simulink model "elevator"  (Simulink 6.5)
settings: Solver=FixedStepDiscrete  StartTime=0.0  StopTime=inf  FixedStep=0.01  RelTol=1e-3
settings Model: Creator=sja  LastModifiedBy=haf  ExtModeAutoUpdateStatusClock=off
settings DebuggingCC: MultiTaskDSMMsg=warning  MultiTaskCondExecSysMsg=none  StrictBusMsg=None
settings RTWCC: IncludeERTFirstTime=on

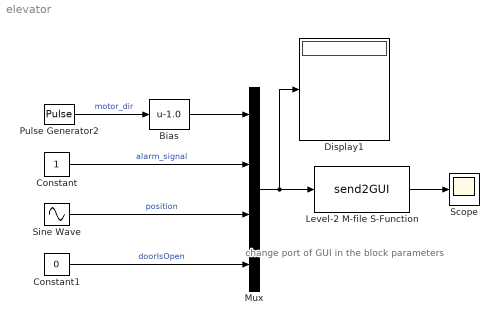
== system elevator ==
  note: change port of
      | GUI in the block
      | parameters
  Bias : Bias  Bias=-1.0
  Constant : Constant  Value=1  OutDataType=sfix(16)  ConRadixGroup=Use specified scaling  OutScaling=2^0  SampleTime=inf  FramePeriod=inf
  Constant1 : Constant  Value=0  OutDataType=sfix(16)  ConRadixGroup=Use specified scaling  OutScaling=2^0  SampleTime=inf  FramePeriod=inf
  Display1 : Display
  Level-2 M-file S-Function : M-S-Function  FunctionName=send2GUI  Parameters=port,dimensions,sampletime  mask{port=1234, dimensions=1, sampletime=-1}
      mask prompts: port "TCP Port for GUI server"; dimensions "Output Port Dimensions"
      mask help: Interface Block to pass data between the model and a graphical user interface accessed via TCP/IP.
      mask init:
      | port = 1234;
      | dimensions = 1;
      | sampletime = -1;
      mask Display:
      | fprintf('GUI INTERFACE\n\n')
      | fprintf(['Port: ' num2str(port)])
  Mux : Mux
  Pulse Generator2 : DiscretePulseGenerator  PulseType=Time based  Amplitude=2  Period=3  PulseWidth=50
  Scope : Scope
      settings: YMin=0.95  YMax=1.05
  Sine Wave : Sin  Amplitude=50  Bias=50  Phase=5  SampleTime=0
  wires:
  Pulse Generator2/1 -> Bias/1  "motor_dir"
  Constant/1 -> Mux/2  "alarm_signal"
  Sine Wave/1 -> Mux/3  "position"
  Constant1/1 -> Mux/4  "doorIsOpen"
  Mux/1 -> Level-2 M-file S-Function/1, Display1/1
  Level-2 M-file S-Function/1 -> Scope/1
  Bias/1 -> Mux/1
